simulink model "UnitTest_relay_InitialConditionMng"  (Simulink 8.1)
settings: Solver=ode45  StartTime=0.0  StopTime=7  RelTol=1e-3
undefined symbols (not defined in the file or in its folder): Initial_cond_mng, relay_tripOutMng_lib
libraries: simulink x4, simulink_extras x1
settings Model: Creator=re25624  LastModifiedBy=re25624
settings DataIOCC: SignalLoggingSaveFormat=Dataset
settings OptimizationCC: ExpressionDepthLimit=128
settings DebuggingCC: FcnCallInpInsideContextMsg=EnableAllAsError
settings GRTTargetCC: CombineOutputUpdateFcns=on  GRTInterface=off

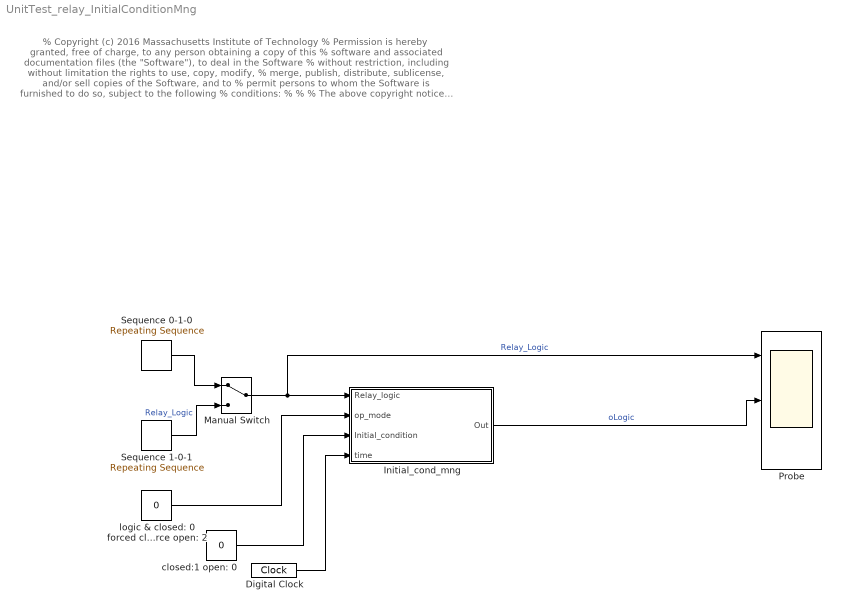
== system UnitTest_relay_InitialConditionMng ==
  note: % Copyright (c) 2016 Massachusetts Institute of Technology
      | % Permission is hereby granted, free of charge, to any person obtaining a copy of this
      | % software and associated documentation files (the "Software"), to deal in the Software
      | % without restriction, including without limitation the rights to use, copy, modify,
      | % merge, publish, distribute, sublicense, and/or sell copies of the Software, and to
      | % permit persons to whom the Software is furnished to do so, subject to the following
      | % conditions:
      | %
      | %
      | % The above copyright notice and this permission notice shall be included in
      | % all copies or substantial portions of the Software.
      | %
      | % THE SOFTWARE IS PROVIDED "AS IS", WITHOUT WARRANTY OF ANY KIND, EXPRESS OR IMPLIED,
      | % INCLUDING BUT NOT LIMITED TO THE WARRANTIES OF MERCHANTABILITY, FITNESS FOR A
      | % PARTICULAR PURPOSE AND NONINFRINGEMENT. IN NO EVENT SHALL THE AUTHORS OR COPYRIGHT
      | % HOLDERS BE LIABLE FOR ANY CLAIM, DAMAGES OR OTHER LIABILITY, WHETHER IN AN ACTION
      | % OF CONTRACT, TORT OR OTHERWISE, ARISING FROM, OUT OF OR IN CONNECTION WITH THE
      | % SOFTWARE OR THE USE OR OTHER DEALINGS IN THE SOFTWARE.
      | %
      | %
      | %%
  Digital Clock : DigitalClock  SampleTime=100e-6
  Initial_cond_mng : Subsystem  AncestorBlock=relay_tripOutMng_lib/Initial_cond_mng
  Manual Switch : ManualSwitch
  Probe : Scope  NumInputPorts=3
      settings: TimeRange=7  YMin=0~0~0  YMax=1.5~1.5~1.5
  Sequence 0-1-0 : simulink/Sources/Repeating Sequence  rep_seq_t=[0 2.5 2.5 4.5 4.5 10]  rep_seq_y=[0 0 1 1 0 0]
  Sequence 1-0-1 : simulink/Sources/Repeating Sequence  rep_seq_t=[0 2.5 2.5 4.5 4.5 10]  rep_seq_y=[1 1 0 0 1 1]
  closed:1 open: 0 : Constant  Value=0
  logic & closed: 0 forced closed: 1 force open: 2 : Constant  Value=0
  wires:
  logic & closed: 0 forced closed: 1 force open: 2/1 -> Initial_cond_mng/2(op_mode)
  closed:1 open: 0/1 -> Initial_cond_mng/3(Initial_condition)
  Digital Clock/1 -> Initial_cond_mng/4(time)
  Manual Switch/1 -> Probe/1, Initial_cond_mng/1(Relay_logic)  "Relay_Logic"
  Initial_cond_mng/1(Out) -> Probe/2  "oLogic"
  ? -> Probe/3  "check Rlogic diff InitCondition"
  Sequence 1-0-1/1 -> Manual Switch/2  "Relay_Logic"
  Sequence 0-1-0/1 -> Manual Switch/1

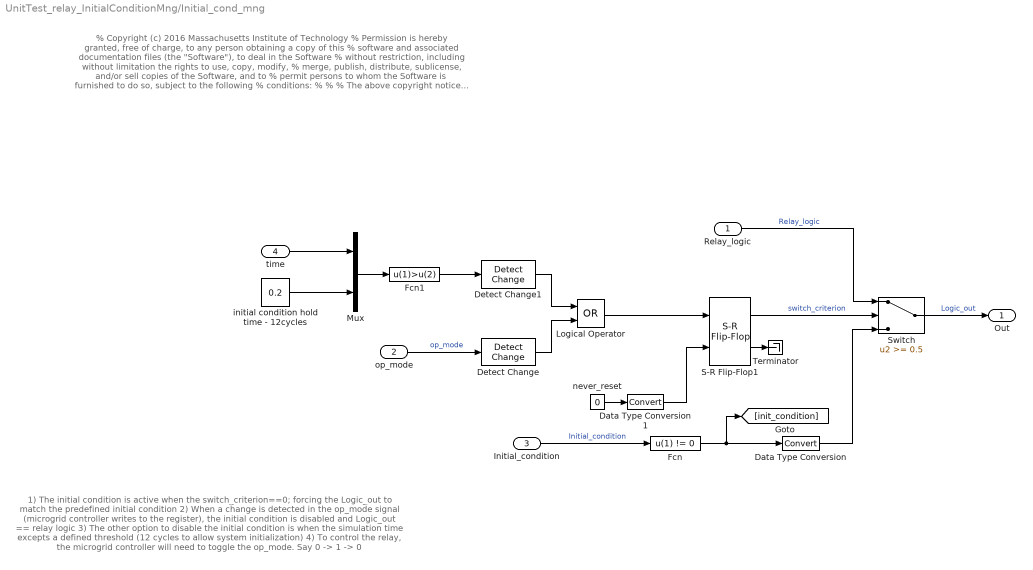
== system UnitTest_relay_InitialConditionMng/Initial_cond_mng ==
  note: 1) The initial condition is active when the switch_criterion==0; forcing the Logic_out to match the predefined initial condition
      | 2) When a change is detected in the op_mode signal (microgrid controller writes to the register), the initial condition is disabled and Logic_out == relay logic
      | 3) The other option to disable the initial condition is when the simulation time excepts a defined threshold (12 cycles to allow system initialization)
      | 4) To control the relay, the microgrid controller will need to toggle the op_mode. Say 0 -> 1 -> 0
  note: % Copyright (c) 2016 Massachusetts Institute of Technology
      | % Permission is hereby granted, free of charge, to any person obtaining a copy of this
      | % software and associated documentation files (the "Software"), to deal in the Software
      | % without restriction, including without limitation the rights to use, copy, modify,
      | % merge, publish, distribute, sublicense, and/or sell copies of the Software, and to
      | % permit persons to whom the Software is furnished to do so, subject to the following
      | % conditions:
      | %
      | %
      | % The above copyright notice and this permission notice shall be included in
      | % all copies or substantial portions of the Software.
      | %
      | % THE SOFTWARE IS PROVIDED "AS IS", WITHOUT WARRANTY OF ANY KIND, EXPRESS OR IMPLIED,
      | % INCLUDING BUT NOT LIMITED TO THE WARRANTIES OF MERCHANTABILITY, FITNESS FOR A
      | % PARTICULAR PURPOSE AND NONINFRINGEMENT. IN NO EVENT SHALL THE AUTHORS OR COPYRIGHT
      | % HOLDERS BE LIABLE FOR ANY CLAIM, DAMAGES OR OTHER LIABILITY, WHETHER IN AN ACTION
      | % OF CONTRACT, TORT OR OTHERWISE, ARISING FROM, OUT OF OR IN CONNECTION WITH THE
      | % SOFTWARE OR THE USE OR OTHER DEALINGS IN THE SOFTWARE.
      | %
      | %
      | %%
  Relay_logic : Inport
  op_mode : Inport  Port=2
  Initial_condition : Inport  Port=3
  time : Inport  Port=4
  Data Type Conversion : DataTypeConversion
  Data Type Conversion1 : DataTypeConversion
  Detect Change : simulink/Logic and Bit Operations/Detect Change  vinit=0  InputProcessing=Inherited  OutDataTypeStr=boolean
  Detect Change1 : simulink/Logic and Bit Operations/Detect Change  vinit=0  InputProcessing=Inherited  OutDataTypeStr=boolean
  Fcn : Fcn  Expr=u(1) != 0
  Fcn1 : Fcn  Expr=u(1)>u(2)
  Logical Operator : Logic  Operator=OR  AllPortsSameDT=off  OutDataTypeStr=boolean
  Mux : Mux  Inputs=2
  S-R Flip-Flop1 : simulink_extras/Flip Flops/S-R Flip-Flop  initial_condition=0
  Switch : Switch  Threshold=0.5
  Terminator : Terminator
  initial condition hold time - 12cycles : Constant  Value=0.2
  never_reset : Constant  Value=0
  Out : Outport
  wires:
  never_reset/1 -> Data Type Conversion1/1
  op_mode/1 -> Detect Change/1  "op_mode"
  Data Type Conversion1/1 -> S-R Flip-Flop1/2
  Switch/1 -> Out/1  "Logic_out"
  S-R Flip-Flop1/2 -> Terminator/1
  S-R Flip-Flop1/1 -> Switch/2  "switch_criterion"
  Fcn/1 -> [init_condition], Data Type Conversion/1
  Initial_condition/1 -> Fcn/1  "Initial_condition"
  Data Type Conversion/1 -> Switch/3
  Relay_logic/1 -> Switch/1  "Relay_logic"
  Mux/1 -> Fcn1/1
  time/1 -> Mux/1
  Fcn1/1 -> Detect Change1/1
  Detect Change1/1 -> Logical Operator/1
  Detect Change/1 -> Logical Operator/2
  Logical Operator/1 -> S-R Flip-Flop1/1
  initial condition hold time - 12cycles/1 -> Mux/2
